simulink model "usb_joystick_testing"  (R2024b)
settings: Solver=VariableStepAuto  StartTime=0.0  StopTime=10.0  RelTol=1e-3
libraries: aerolibanimutils x2
settings Model: Creator=conno  LastModifiedBy=conno

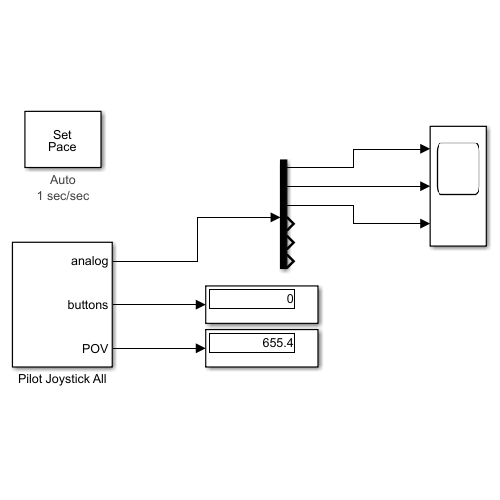
[thumbnail: Simulink's stored preview of the top-level diagram]
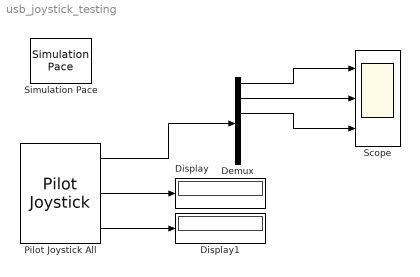
== system usb_joystick_testing ==
  Demux : Demux  Outputs=6
  Display : Display
  Display1 : Display
  Pilot Joystick All : aerolibanimutils/Pilot Joystick  JoystickID=Joystick1  OutputConfiguration=AllOutputs  SampleTime=1/50
      settings: LibrarySourceBlock=aerolibanimutils/Pilot Joystick All
  Scope : Scope  NumInputPorts=3
  Simulation Pace : aerolibanimutils/Simulation Pace  SimulationPace=1  SleepMode=Auto  OutputPaceError=off  SampleTime=1/50
  wires:
  Pilot Joystick All/1 -> Demux/1
  Demux/2 -> Scope/2
  Pilot Joystick All/3 -> Display1/1
  Demux/3 -> Scope/3
  Pilot Joystick All/2 -> Display/1
  Demux/1 -> Scope/1
